simulink model "Assem2"  (R2017a)
settings: Solver=ode5  StartTime=0.0  StopTime=T  FixedStep=0.01  RelTol=1e-3
values from neighbouring files (symbols this model uses):
  N = 30    [movC.m]    (also in movC_smooth.m = 60; movL.m; rotX.m; something.m = 50000)
undefined symbols (not defined in the file or in its folder): base, link1, link2, link3, link4
libraries: mblibv1 x18, simulink x4
settings Model: Creator=Admin  LastModifiedBy=Admin
settings SimMechanicsCC: VisOnUpdateDiagram=on  VisDuringSimulation=on

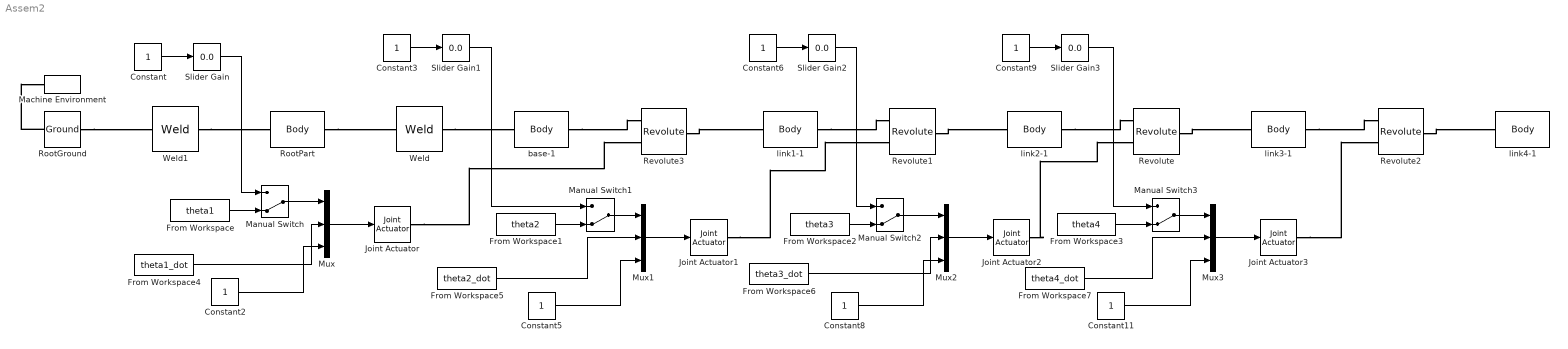
== system Assem2 ==
  Constant{,2..3,5..6,8..9,11} (8 alike) : Constant
  From Workspace : FromWorkspace  VariableName=theta1  SampleTime=0  OutputAfterFinalValue=Holding final value
  From Workspace1 : FromWorkspace  VariableName=theta2  SampleTime=0  OutputAfterFinalValue=Holding final value
  From Workspace2 : FromWorkspace  VariableName=theta3  SampleTime=0  OutputAfterFinalValue=Holding final value
  From Workspace3 : FromWorkspace  VariableName=theta4  SampleTime=0  OutputAfterFinalValue=Holding final value
  From Workspace4 : FromWorkspace  VariableName=theta1_dot  SampleTime=0  OutputAfterFinalValue=Holding final value
  From Workspace5 : FromWorkspace  VariableName=theta2_dot  SampleTime=0  OutputAfterFinalValue=Holding final value
  From Workspace6 : FromWorkspace  VariableName=theta3_dot  SampleTime=0  OutputAfterFinalValue=Holding final value
  From Workspace7 : FromWorkspace  VariableName=theta4_dot  SampleTime=0  OutputAfterFinalValue=Holding final value
  Joint Actuator{,1..3} (4 alike) : mblibv1/Sensors &  Actuators/Joint Actuator  UpdateFromCAD=off  PhysicalDomain=Mechanical  PortType=blob  ActuationStyle=Motion  AngleUnits=deg  ArcVelocityUnits=deg/s  ArcAccelerationUnits=deg/s^2  CoordPositionUnits=m  VelocityUnits=m/s  AccelerationUnits=m/s^2  ForceUnits=N  TorqueUnits=N*m  ActiveIO=on  Width=3  DialogClass=MechanicalActuatorBlock  Primitive=R1  ReferenceFrame=Absolute (World)
      settings: SourceProductName=Simscape Multibody  SourceProductBaseCode=MS
  Machine Environment : mblibv1/Bodies/Machine Environment  PortType=env  PhysicalDomain=Mechanical  DialogTemplateClass=MECH.MachineEnvironment  SyncWhenCopied=off  Gravity=[0 -9.81 0]  GravityUnits=m/s^2  GravityAsSignal=off  Dimensionality=Auto-detect  AnalysisType=Forward dynamics  LinearAssemblyTolerance=1e-3  LinearAssemblyToleranceUnits=m  AngularAssemblyTolerance=1e-3  AngularAssemblyToleranceUnits=rad  ConstraintSolverType=Stabilizing  ConstraintRelTolerance=1e-4  ConstraintAbsTolerance=1e-4  UseRobustSingularityHandling=off  RedundancyAnalysisToleranceType=Automatically select tolerance  RedundancyAnalysisTolerance=1e-14  StatePerturbationType=Fixed  PerturbationSize=1e-5  VisualizeMachine=on  BodyVisualizationType=Use model default body geometries  BodyColorSelMode=Use model default  DefaultBodyColor=[1 0 0]
      settings: SourceProductName=Simscape Multibody  SourceProductBaseCode=MS
  Manual Switch{,1..3} (4 alike) : ManualSwitch  CurrentSetting=0
  Mux{,1..3} (4 alike) : Mux  Inputs=3
  Revolute : mblibv1/Joints/Revolute  LConnTagsString=__newl0|SA1  RConnTagsString=__newr0  UpdateFromCAD=on  PMImportedID=link2-1:-:link3-1  NumSAPorts=1  CutJoint=off  MarkAsCut=off  Primitives=prismatic  PrimitiveProps=R1$World$[0,-1,0]$revolute  DialogClass=JointBlock  R1Axis=[0,-1,0]
      settings: SourceProductName=Simscape Multibody  SourceProductBaseCode=MS
  Revolute1 : mblibv1/Joints/Revolute  LConnTagsString=__newl0|SA1  RConnTagsString=__newr0  UpdateFromCAD=on  PMImportedID=link1-1:-:link2-1  NumSAPorts=1  CutJoint=off  MarkAsCut=off  Primitives=prismatic  PrimitiveProps=R1$World$[0,-1,0]$revolute  DialogClass=JointBlock  R1Axis=[0,-1,0]
      settings: SourceProductName=Simscape Multibody  SourceProductBaseCode=MS
  Revolute2 : mblibv1/Joints/Revolute  LConnTagsString=__newl0|SA1  RConnTagsString=__newr0  UpdateFromCAD=on  PMImportedID=link3-1:-:link4-1  NumSAPorts=1  CutJoint=off  MarkAsCut=off  Primitives=prismatic  PrimitiveProps=R1$World$[0,1,0]$revolute  DialogClass=JointBlock  R1Axis=[0,1,0]
      settings: SourceProductName=Simscape Multibody  SourceProductBaseCode=MS
  Revolute3 : mblibv1/Joints/Revolute  LConnTagsString=__newl0|SA1  RConnTagsString=__newr0  UpdateFromCAD=on  PMImportedID=base-1:-:link1-1  NumSAPorts=1  CutJoint=off  MarkAsCut=off  Primitives=prismatic  PrimitiveProps=R1$World$[0,0,1]$revolute  DialogClass=JointBlock  R1Axis=[0,0,1]
      settings: SourceProductName=Simscape Multibody  SourceProductBaseCode=MS
  RootGround : mblibv1/Bodies/Ground  UpdateFromCAD=on  PMImportedID=RootGround  LeftPortType=env  RightPortType=workingframe  PhysicalDomain=Mechanical  DialogClass=GroundBlock  CoordPosition=[0.0706023,0.00354461,0.184253]  CoordPositionUnits=m  StateVectorMgrId=0  MachineId=[1 0]  ShowEnvPort=on  ParameterChecksum=[1441791627, 2887137816, 2946438640, 4094387026]  TopologyChecksum=[3009767189, 3815855394, 2415198278, 2816644252]
      settings: SourceProductName=Simscape Multibody  SourceProductBaseCode=MS
  RootPart : mblibv1/Bodies/Body  LConnTagsString=CS3  RConnTagsString=CS2  UpdateFromCAD=on  PMImportedID=Assem2/RootPart  DialogClass=MechanicalBodyBlock  Mass=0  MassUnits=kg  InertiaUnits=kg*m^2  Inertia=[0,0,0;0,0,0;0,0,0]  Shape=Cylinder  ShapeDims=[1 1]  ShapeUnits=m  ShapeUse=false  Density=1  DensityUnits=kg/m^3  DensityUse=false  GraphicsMode=MACHINE_DEFAULT  BodyColorSelMode=MACHINE_DEFAULT  BodyColor=[1;0;0]  AttachedToCS=CS1  CG=Right$CG$[0.0706023 0.00354461 0.184253]$WORLD$WORLD$m$[1 0 0;0 1 0;0 0 1]$3x3 Transform$rad$WORLD$false$Assem2/RootPart::CG(AUTOGEN)  WorkingFrames=Right$CS1$[0 0 0]$WORLD$WORLD$m$[1 0 0;0 1 0;0 0 1]$3x3 Transform$rad$WORLD$false$Assem2/RootPart::CS1(AUTOGEN)#Right$CS2$[-0.0347872 0.00354461 0.0459347]$WORLD$WORLD$m$[1 0 0;0 1 0;0 0 1]$3x3 Transform$rad$WORLD$true$Assem2/RootPart:-:base-1::Assem2/RootPart(AUTOGEN)#Left$CS3$[0.0706023 0.00354461 0.184253]$WORLD$WORLD$m$[1 0 0;0 1 0;0 0 1]$3x3 Transform$rad$WORLD$true$Assem2/RootPart:-:RootGround::Assem2/RootPart(AUTOGEN)  CGPos=[0.0706023 0.00354461 0.184253]  CGRot=[1 0 0;0 1 0;0 0 1]  CS0Pos=[]  CS0Rot=[]  CS1Pos=[0 0 0]  CS1Rot=[1 0 0;0 1 0;0 0 1]  CS2Pos=[-0.0347872 0.00354461 0.0459347]  CS2Rot=[1 0 0;0 1 0;0 0 1]  CS3Pos=[0.0706023 0.00354461 0.184253]  CS3Rot=[1 0 0;0 1 0;0 0 1]  CS4Pos=[]  CS4Rot=[]  CS5Pos=[]  CS5Rot=[]  CS6Pos=[]  CS6Rot=[]  CS7Pos=[]  CS7Rot=[]  CS8Pos=[]  CS8Rot=[]  CS9Pos=[]  CS9Rot=[]  CS10Pos=[]  CS10Rot=[]  CS11Pos=[]  CS11Rot=[]  CS12Pos=[]  CS12Rot=[]  CS13Pos=[]  CS13Rot=[]  CS14Pos=[]  CS14Rot=[]  CS15Pos=[]  CS15Rot=[]  CS16Pos=[]  CS16Rot=[]  CS17Pos=[]  CS17Rot=[]  CS18Pos=[]  CS18Rot=[]  CS19Pos=[]  CS19Rot=[]  CS20Pos=[]  CS20Rot=[]
      settings: SourceProductName=Simscape Multibody  SourceProductBaseCode=MS
  Slider Gain : simulink/Math Operations/Slider Gain  gain=0.0  low=0  high=180
  Slider Gain1 : simulink/Math Operations/Slider Gain  gain=0.0  low=-180  high=180
  Slider Gain2 : simulink/Math Operations/Slider Gain  gain=0.0  low=0  high=180
  Slider Gain3 : simulink/Math Operations/Slider Gain  gain=0.0  low=0  high=180
  Weld : mblibv1/Joints/Weld  LConnTagsString=__newl0  RConnTagsString=__newr0  UpdateFromCAD=on  PMImportedID=Assem2/RootPart:-:base-1  NumSAPorts=0  CutJoint=off  MarkAsCut=off  Primitives=weld  PrimitiveProps=W$WORLD$[0.57735,0.57735,0.57735]$weld  DialogClass=JointBlock  WAxis=[0.57735,0.57735,0.57735]
      settings: SourceProductName=Simscape Multibody  SourceProductBaseCode=MS
  Weld1 : mblibv1/Joints/Weld  LConnTagsString=__newl0  RConnTagsString=__newr0  UpdateFromCAD=on  PMImportedID=Assem2/RootPart:-:RootGround  NumSAPorts=0  CutJoint=off  MarkAsCut=off  Primitives=weld  PrimitiveProps=W$WORLD$[0.57735,0.57735,0.57735]$weld  DialogClass=JointBlock  WAxis=[0.57735,0.57735,0.57735]
      settings: SourceProductName=Simscape Multibody  SourceProductBaseCode=MS
  base-1 : mblibv1/Bodies/Body  LConnTagsString=CS2  RConnTagsString=CS3  UpdateFromCAD=on  PMImportedID=base-1  DialogClass=MechanicalBodyBlock  Mass=0.0547939  MassUnits=kg  InertiaUnits=kg*m^2  Inertia=[1.07468e-05,0,-2.78582e-07;0,1.65699e-05,0;-2.78582e-07,0,1.64257e-05]  Shape=Cylinder  ShapeDims=[1 1]  ShapeUnits=m  ShapeUse=false  Density=1  DensityUnits=kg/m^3  DensityUse=false  GraphicsMode=GFXFILE  GraphicsFileName=Assem2 - base-1.STL  BodyColorSelMode=COLORPALETTE  BodyColor=[0.215686;0.619608;1]  AttachedToCS=CS1  CG=Right$CG$[-0.0347872 0.00354461 0.0459347]$WORLD$WORLD$m$[1 0 0;0 1 0;0 0 1]$3x3 Transform$rad$WORLD$false$base-1::CG(AUTOGEN)  WorkingFrames=Right$CS1$[-0.0240069 0.00354461 0.069]$WORLD$WORLD$m$[1 0 0;0 1 0;0 0 1]$3x3 Transform$rad$WORLD$false$base-1::CS1(AUTOGEN)#Left$CS2$[-0.0347872 0.00354461 0.0459347]$WORLD$WORLD$m$[1 0 0;0 1 0;0 0 1]$3x3 Transform$rad$WORLD$true$Assem2/RootPart:-:base-1::base-1(AUTOGEN)#Right$CS3$[-0.0240069 0.00354461 0.066]$WORLD$WORLD$m$[1 0 0;0 1 0;0 0 1]$3x3 Transform$rad$WORLD$true$base-1:-:link1-1::base-1(AUTOGEN)  CGPos=[-0.0347872 0.00354461 0.0459347]  CGRot=[1 0 0;0 1 0;0 0 1]  CS0Pos=[]  CS0Rot=[]  CS1Pos=[-0.0240069 0.00354461 0.069]  CS1Rot=[1 0 0;0 1 0;0 0 1]  CS2Pos=[-0.0347872 0.00354461 0.0459347]  CS2Rot=[1 0 0;0 1 0;0 0 1]  CS3Pos=[-0.0240069 0.00354461 0.066]  CS3Rot=[1 0 0;0 1 0;0 0 1]  CS4Pos=[]  CS4Rot=[]  CS5Pos=[]  CS5Rot=[]  CS6Pos=[]  CS6Rot=[]  CS7Pos=[]  CS7Rot=[]  CS8Pos=[]  CS8Rot=[]  CS9Pos=[]  CS9Rot=[]  CS10Pos=[]  CS10Rot=[]  CS11Pos=[]  CS11Rot=[]  CS12Pos=[]  CS12Rot=[]  CS13Pos=[]  CS13Rot=[]  CS14Pos=[]  CS14Rot=[]  CS15Pos=[]  CS15Rot=[]  CS16Pos=[]  CS16Rot=[]  CS17Pos=[]  CS17Rot=[]  CS18Pos=[]  CS18Rot=[]  CS19Pos=[]  CS19Rot=[]  CS20Pos=[]  CS20Rot=[]
      settings: SourceProductName=Simscape Multibody  SourceProductBaseCode=MS
  link1-1 : mblibv1/Bodies/Body  LConnTagsString=CS3  RConnTagsString=CS2  UpdateFromCAD=on  PMImportedID=link1-1  DialogClass=MechanicalBodyBlock  Mass=0.0553342  MassUnits=kg  InertiaUnits=kg*m^2  Inertia=[1.8235e-05,0,0;0,1.05975e-05,0;0,0,1.53152e-05]  Shape=Cylinder  ShapeDims=[1 1]  ShapeUnits=m  ShapeUse=false  Density=1  DensityUnits=kg/m^3  DensityUse=false  GraphicsMode=GFXFILE  GraphicsFileName=Assem2 - link1-1.STL  BodyColorSelMode=COLORPALETTE  BodyColor=[0.792157;0.819608;0.933333]  AttachedToCS=CS1  CG=Right$CG$[-0.0240069 0.00354461 0.0918404]$WORLD$WORLD$m$[1 0 0;0 0 -1;0 1 0]$3x3 Transform$rad$WORLD$false$link1-1::CG(AUTOGEN)  WorkingFrames=Right$CS1$[-0.0240069 0.00354461 0.104]$WORLD$WORLD$m$[1 0 0;0 0 -1;0 1 0]$3x3 Transform$rad$WORLD$false$link1-1::CS1(AUTOGEN)#Right$CS2$[-0.0240069 -0.0204554 0.104]$WORLD$WORLD$m$[1 0 0;0 1 0;0 0 1]$3x3 Transform$rad$WORLD$true$link1-1:-:link2-1::link1-1(AUTOGEN)#Left$CS3$[-0.0240069 0.00354461 0.066]$WORLD$WORLD$m$[1 0 0;0 1 0;0 0 1]$3x3 Transform$rad$WORLD$true$base-1:-:link1-1::link1-1(AUTOGEN)  CGPos=[-0.0240069 0.00354461 0.0918404]  CGRot=[1 0 0;0 0 -1;0 1 0]  CS0Pos=[]  CS0Rot=[]  CS1Pos=[-0.0240069 0.00354461 0.104]  CS1Rot=[1 0 0;0 0 -1;0 1 0]  CS2Pos=[-0.0240069 -0.0204554 0.104]  CS2Rot=[1 0 0;0 1 0;0 0 1]  CS3Pos=[-0.0240069 0.00354461 0.066]  CS3Rot=[1 0 0;0 1 0;0 0 1]  CS4Pos=[]  CS4Rot=[]  CS5Pos=[]  CS5Rot=[]  CS6Pos=[]  CS6Rot=[]  CS7Pos=[]  CS7Rot=[]  CS8Pos=[]  CS8Rot=[]  CS9Pos=[]  CS9Rot=[]  CS10Pos=[]  CS10Rot=[]  CS11Pos=[]  CS11Rot=[]  CS12Pos=[]  CS12Rot=[]  CS13Pos=[]  CS13Rot=[]  CS14Pos=[]  CS14Rot=[]  CS15Pos=[]  CS15Rot=[]  CS16Pos=[]  CS16Rot=[]  CS17Pos=[]  CS17Rot=[]  CS18Pos=[]  CS18Rot=[]  CS19Pos=[]  CS19Rot=[]  CS20Pos=[]  CS20Rot=[]
      settings: SourceProductName=Simscape Multibody  SourceProductBaseCode=MS
  link2-1 : mblibv1/Bodies/Body  LConnTagsString=CS3  RConnTagsString=CS2  UpdateFromCAD=on  PMImportedID=link2-1  DialogClass=MechanicalBodyBlock  Mass=0.117048  MassUnits=kg  InertiaUnits=kg*m^2  Inertia=[0.000233359,-2.83101e-05,0;-2.83101e-05,3.2542e-05,0;0,0,0.00023539]  Shape=Cylinder  ShapeDims=[1 1]  ShapeUnits=m  ShapeUse=false  Density=1  DensityUnits=kg/m^3  DensityUse=false  GraphicsMode=GFXFILE  GraphicsFileName=Assem2 - link2-1.STL  BodyColorSelMode=COLORPALETTE  BodyColor=[0.792157;0.819608;0.933333]  AttachedToCS=CS1  CG=Right$CG$[-0.0181758 0.00354461 0.190521]$WORLD$WORLD$m$[1 0 0;0 0 -1;0 1 0]$3x3 Transform$rad$WORLD$false$link2-1::CG(AUTOGEN)  WorkingFrames=Right$CS1$[-6.85388e-06 0.00354461 0.232]$WORLD$WORLD$m$[1 0 0;0 0 -1;0 1 0]$3x3 Transform$rad$WORLD$false$link2-1::CS1(AUTOGEN)#Right$CS2$[-6.85388e-06 0.0267946 0.232]$WORLD$WORLD$m$[1 0 0;0 1 0;0 0 1]$3x3 Transform$rad$WORLD$true$link2-1:-:link3-1::link2-1(AUTOGEN)#Left$CS3$[-0.0240069 -0.0204554 0.104]$WORLD$WORLD$m$[1 0 0;0 1 0;0 0 1]$3x3 Transform$rad$WORLD$true$link1-1:-:link2-1::link2-1(AUTOGEN)  CGPos=[-0.0181758 0.00354461 0.190521]  CGRot=[1 0 0;0 0 -1;0 1 0]  CS0Pos=[]  CS0Rot=[]  CS1Pos=[-6.85388e-06 0.00354461 0.232]  CS1Rot=[1 0 0;0 0 -1;0 1 0]  CS2Pos=[-6.85388e-06 0.0267946 0.232]  CS2Rot=[1 0 0;0 1 0;0 0 1]  CS3Pos=[-0.0240069 -0.0204554 0.104]  CS3Rot=[1 0 0;0 1 0;0 0 1]  CS4Pos=[]  CS4Rot=[]  CS5Pos=[]  CS5Rot=[]  CS6Pos=[]  CS6Rot=[]  CS7Pos=[]  CS7Rot=[]  CS8Pos=[]  CS8Rot=[]  CS9Pos=[]  CS9Rot=[]  CS10Pos=[]  CS10Rot=[]  CS11Pos=[]  CS11Rot=[]  CS12Pos=[]  CS12Rot=[]  CS13Pos=[]  CS13Rot=[]  CS14Pos=[]  CS14Rot=[]  CS15Pos=[]  CS15Rot=[]  CS16Pos=[]  CS16Rot=[]  CS17Pos=[]  CS17Rot=[]  CS18Pos=[]  CS18Rot=[]  CS19Pos=[]  CS19Rot=[]  CS20Pos=[]  CS20Rot=[]
      settings: SourceProductName=Simscape Multibody  SourceProductBaseCode=MS
  link3-1 : mblibv1/Bodies/Body  LConnTagsString=CS2  RConnTagsString=CS3  UpdateFromCAD=on  PMImportedID=link3-1  DialogClass=MechanicalBodyBlock  Mass=0.0869839  MassUnits=kg  InertiaUnits=kg*m^2  Inertia=[1.69409e-05,0,0;0,0.000140539,0;0,0,0.000129904]  Shape=Cylinder  ShapeDims=[1 1]  ShapeUnits=m  ShapeUse=false  Density=1  DensityUnits=kg/m^3  DensityUse=false  GraphicsMode=GFXFILE  GraphicsFileName=Assem2 - link3-1.STL  BodyColorSelMode=COLORPALETTE  BodyColor=[1;0.298039;0.184314]  AttachedToCS=CS1  CG=Right$CG$[0.0749366 0.00354461 0.232]$WORLD$WORLD$m$[1 0 0;0 0 -1;0 1 0]$3x3 Transform$rad$WORLD$false$link3-1::CG(AUTOGEN)  WorkingFrames=Right$CS1$[0.123993 0.00354461 0.232]$WORLD$WORLD$m$[1 0 0;0 0 -1;0 1 0]$3x3 Transform$rad$WORLD$false$link3-1::CS1(AUTOGEN)#Left$CS2$[-6.85388e-06 0.0267946 0.232]$WORLD$WORLD$m$[1 0 0;0 1 0;0 0 1]$3x3 Transform$rad$WORLD$true$link2-1:-:link3-1::link3-1(AUTOGEN)#Right$CS3$[0.123993 0.0267946 0.232]$WORLD$WORLD$m$[1 0 0;0 1 0;0 0 1]$3x3 Transform$rad$WORLD$true$link3-1:-:link4-1::link3-1(AUTOGEN)  CGPos=[0.0749366 0.00354461 0.232]  CGRot=[1 0 0;0 0 -1;0 1 0]  CS0Pos=[]  CS0Rot=[]  CS1Pos=[0.123993 0.00354461 0.232]  CS1Rot=[1 0 0;0 0 -1;0 1 0]  CS2Pos=[-6.85388e-06 0.0267946 0.232]  CS2Rot=[1 0 0;0 1 0;0 0 1]  CS3Pos=[0.123993 0.0267946 0.232]  CS3Rot=[1 0 0;0 1 0;0 0 1]  CS4Pos=[]  CS4Rot=[]  CS5Pos=[]  CS5Rot=[]  CS6Pos=[]  CS6Rot=[]  CS7Pos=[]  CS7Rot=[]  CS8Pos=[]  CS8Rot=[]  CS9Pos=[]  CS9Rot=[]  CS10Pos=[]  CS10Rot=[]  CS11Pos=[]  CS11Rot=[]  CS12Pos=[]  CS12Rot=[]  CS13Pos=[]  CS13Rot=[]  CS14Pos=[]  CS14Rot=[]  CS15Pos=[]  CS15Rot=[]  CS16Pos=[]  CS16Rot=[]  CS17Pos=[]  CS17Rot=[]  CS18Pos=[]  CS18Rot=[]  CS19Pos=[]  CS19Rot=[]  CS20Pos=[]  CS20Rot=[]
      settings: SourceProductName=Simscape Multibody  SourceProductBaseCode=MS
  link4-1 : mblibv1/Bodies/Body  LConnTagsString=CS2  UpdateFromCAD=on  PMImportedID=link4-1  DialogClass=MechanicalBodyBlock  Mass=0.16348  MassUnits=kg  InertiaUnits=kg*m^2  Inertia=[0.000112546,0,0;0,0.000266976,0;0,0,0.000183011]  Shape=Cylinder  ShapeDims=[1 1]  ShapeUnits=m  ShapeUse=false  Density=1  DensityUnits=kg/m^3  DensityUse=false  GraphicsMode=GFXFILE  GraphicsFileName=Assem2 - link4-1.STL  BodyColorSelMode=COLORPALETTE  BodyColor=[0.792157;0.819608;0.933333]  AttachedToCS=CS1  CG=Right$CG$[0.199206 0.00354461 0.232]$WORLD$WORLD$m$[1 0 0;0 0 -1;0 1 0]$3x3 Transform$rad$WORLD$false$link4-1::CG(AUTOGEN)  WorkingFrames=Right$CS1$[0.249993 0.00354461 0.232]$WORLD$WORLD$m$[1 0 0;0 0 -1;0 1 0]$3x3 Transform$rad$WORLD$false$link4-1::CS1(AUTOGEN)#Left$CS2$[0.123993 0.0267946 0.232]$WORLD$WORLD$m$[1 0 0;0 1 0;0 0 1]$3x3 Transform$rad$WORLD$true$link3-1:-:link4-1::link4-1(AUTOGEN)  CGPos=[0.199206 0.00354461 0.232]  CGRot=[1 0 0;0 0 -1;0 1 0]  CS0Pos=[]  CS0Rot=[]  CS1Pos=[0.249993 0.00354461 0.232]  CS1Rot=[1 0 0;0 0 -1;0 1 0]  CS2Pos=[0.123993 0.0267946 0.232]  CS2Rot=[1 0 0;0 1 0;0 0 1]  CS3Pos=[]  CS3Rot=[]  CS4Pos=[]  CS4Rot=[]  CS5Pos=[]  CS5Rot=[]  CS6Pos=[]  CS6Rot=[]  CS7Pos=[]  CS7Rot=[]  CS8Pos=[]  CS8Rot=[]  CS9Pos=[]  CS9Rot=[]  CS10Pos=[]  CS10Rot=[]  CS11Pos=[]  CS11Rot=[]  CS12Pos=[]  CS12Rot=[]  CS13Pos=[]  CS13Rot=[]  CS14Pos=[]  CS14Rot=[]  CS15Pos=[]  CS15Rot=[]  CS16Pos=[]  CS16Rot=[]  CS17Pos=[]  CS17Rot=[]  CS18Pos=[]  CS18Rot=[]  CS19Pos=[]  CS19Rot=[]  CS20Pos=[]  CS20Rot=[]
      settings: SourceProductName=Simscape Multibody  SourceProductBaseCode=MS
  wires:
  Mux/1 -> Joint Actuator/1
  Constant2/1 -> Mux/3
  Constant5/1 -> Mux1/3
  From Workspace5/1 -> Mux1/2
  Mux1/1 -> Joint Actuator1/1
  Mux2/1 -> Joint Actuator2/1
  From Workspace6/1 -> Mux2/2
  Constant8/1 -> Mux2/3
  Constant11/1 -> Mux3/3
  From Workspace7/1 -> Mux3/2
  Mux3/1 -> Joint Actuator3/1
  Constant/1 -> Slider Gain/1
  Manual Switch/1 -> Mux/1
  Manual Switch1/1 -> Mux1/1
  Manual Switch2/1 -> Mux2/1
  Manual Switch3/1 -> Mux3/1
  From Workspace3/1 -> Manual Switch3/2
  From Workspace2/1 -> Manual Switch2/2
  From Workspace1/1 -> Manual Switch1/2
  From Workspace/1 -> Manual Switch/2
  Constant3/1 -> Slider Gain1/1
  Constant6/1 -> Slider Gain2/1
  Constant9/1 -> Slider Gain3/1
  Slider Gain3/1 -> Manual Switch3/1
  Slider Gain2/1 -> Manual Switch2/1
  Slider Gain1/1 -> Manual Switch1/1
  Slider Gain/1 -> Manual Switch/1
  From Workspace4/1 -> Mux/2
  connections:
  RootPart/RConn1 -- Weld/LConn1
  Weld/RConn1 -- base-1/LConn1
  link2-1/RConn1 -- Revolute/LConn1
  Revolute/RConn1 -- link3-1/LConn1
  link1-1/RConn1 -- Revolute1/LConn1
  Revolute1/RConn1 -- link2-1/LConn1
  link3-1/RConn1 -- Revolute2/LConn1
  Revolute2/RConn1 -- link4-1/LConn1
  base-1/RConn1 -- Revolute3/LConn1
  Revolute3/RConn1 -- link1-1/LConn1
  RootGround/RConn1 -- Weld1/LConn1
  Weld1/RConn1 -- RootPart/LConn1
  RootGround/LConn1 -- Machine Environment/RConn1
  Joint Actuator/RConn1 -- Revolute3/LConn2
  Joint Actuator1/RConn1 -- Revolute1/LConn2
  Joint Actuator2/RConn1 -- Revolute/LConn2
  Joint Actuator3/RConn1 -- Revolute2/LConn2
